simulink model "RPC_state_feedback"  (R2016b)
settings: Solver=ode45  StartTime=0.0  StopTime=100  RelTol=1e-3  EnableMultiTasking=on
values from neighbouring files (symbols this model uses):
  G = Kp*Kv/s/(s+Kv)    [RPC_script.m]
undefined symbols (not defined in the file or in its folder): A, B, C, D, Fes, K, L
libraries: simulink x2
settings Model: Creator=oboe  LastModifiedBy=oboe
settings DataIOCC: LimitDataPoints=on  SaveFormat=Array
settings OptimizationCC: LifeSpan=inf
settings DebuggingCC: SolverPrmCheckMsg=warning  SFUnexpectedBacktrackingDiag=warning  SFNoUnconditionalDefaultTransitionDiag=warning  SFExecutionAtInitializationDiag=none
settings HardwareCC: ProdBitPerPointer=32  ProdBitPerSizeT=32  ProdBitPerPtrDiffT=32  ProdLargestAtomicFloat=None  ProdIntDivRoundTo=Undefined  ProdEndianess=Unspecified  ProdWordSize=32  ProdHWDeviceType=32-bit Generic
settings ModelReferenceCC: PropagateSignalLabelsOutOfModel=off
settings GRTTargetCC: TargetLangStandard=C89/C90 (ANSI)  GeneratePreprocessorConditionals=Disable all
settings ConfigComp: CovMetricSettings=dw  CovHtmlReporting=on  CovSaveCumulativeToWorkspaceVar=on  CovSaveSingleToWorkspaceVar=on  CovExternalEMLEnable=off  CovSFcnEnable=off

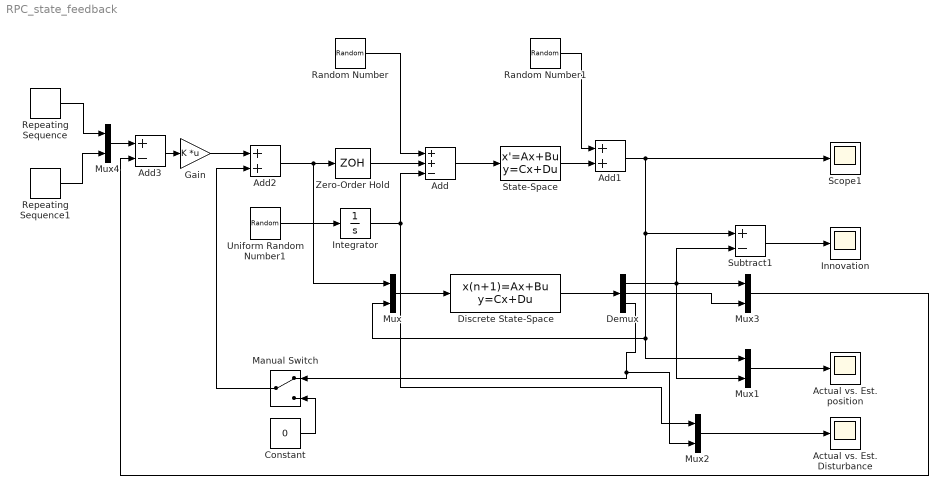
== system RPC_state_feedback ==
  Actual vs. Est. Disturbance : Scope
  Actual vs. Est. position : Scope
  Add : Sum  Inputs=++-
  Add1 : Sum
  Add2 : Sum
  Add3 : Sum  Inputs=+-
  Constant : Constant  Value=0
  Demux : Demux  Outputs=3
  Discrete State-Space : DiscreteStateSpace  A=Fes  B=[G L]  C=eye(3)  D=zeros(3,2)  SampleTime=.001
  Gain : Gain  Gain=K  Multiplication=Matrix(K*u)
  Innovation : Scope
  Integrator : Integrator
  Manual Switch : ManualSwitch
  Mux{,1..4} (5 alike) : Mux  Inputs=2
  Random Number : RandomNumber  Variance=(10/2^12)^2/12  SampleTime=0.001
  Random Number1 : RandomNumber  Variance=(2*pi/2000)^2/12  Seed=124  SampleTime=0.001
  Repeating Sequence : simulink/Sources/Repeating Sequence  rep_seq_t=[0 1 2 3 4]  rep_seq_y=[0 0 1 1 0]
  Repeating Sequence1 : simulink/Sources/Repeating Sequence  rep_seq_t=[0 1-0.001 1 2-0.001 2 3-0.001 3 4-0.001 4]  rep_seq_y=[0 0 1 1 0 0 -1 -1 0]
  Scope1 : Scope
  State-Space : StateSpace  A=A  B=B  C=C  D=D  X0=0
  Subtract1 : Sum  Inputs=+-
  Uniform Random Number1 : UniformRandomNumber  Seed=50  SampleTime=0.001
  Zero-Order Hold : ZeroOrderHold  SampleTime=0.001
  wires:
  Mux/1 -> Discrete State-Space/1
  Discrete State-Space/1 -> Demux/1
  Demux/1 -> Mux3/1, Mux1/2, Subtract1/2
  Mux1/1 -> Actual vs. Est. position/1
  Add/1 -> State-Space/1
  Subtract1/1 -> Innovation/1
  Random Number1/1 -> Add1/1
  Add1/1 -> Mux/2, Mux1/1, Subtract1/1, Scope1/1
  Zero-Order Hold/1 -> Add/2
  Random Number/1 -> Add/1
  State-Space/1 -> Add1/2
  Integrator/1 -> Mux2/1, Add/3
  Uniform Random Number1/1 -> Integrator/1
  Gain/1 -> Add2/1
  Add2/1 -> Mux/1, Zero-Order Hold/1
  Demux/3 -> Manual Switch/1, Mux2/2
  Mux2/1 -> Actual vs. Est. Disturbance/1
  Demux/2 -> Mux3/2
  Repeating Sequence/1 -> Mux4/1
  Repeating Sequence1/1 -> Mux4/2
  Mux4/1 -> Add3/1
  Mux3/1 -> Add3/2
  Add3/1 -> Gain/1
  Manual Switch/1 -> Add2/2
  Constant/1 -> Manual Switch/2
